simulink subsystem "PIDFeedFowardDigital_SubSystem"  (R2020b)
settings: Solver=VariableStepAuto  StartTime=0.0  StopTime=10.0  RelTol=1e-3
values from neighbouring files (symbols this model uses):
  Beq = BeqEst    [loadParNominal.m]
  Jeq = mot.J+(mld.J/gbox.N1^2)    [loadParNominal.m]
  Req = mot.R + sens.curr.Rs    [loadParNominal.m]
undefined symbols (not defined in the file or in its folder): drv, gbox, mld, mot
settings Model: Creator=umbe  LastModifiedBy=umbe

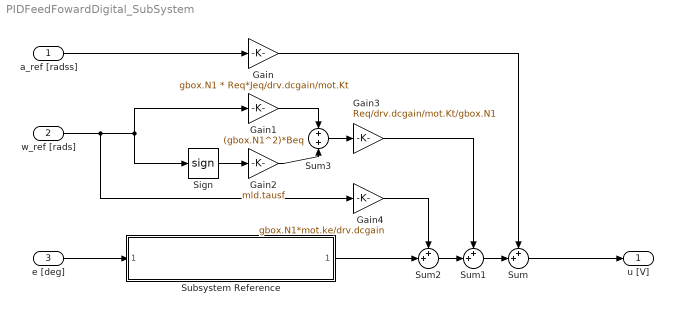
== system PIDFeedFowardDigital_SubSystem ==
  a_ref [radss] : Inport
  w_ref [rads] : Inport  Port=2
  e [deg] : Inport  Port=3
  Gain : Gain  Gain=gbox.N1 * Req*Jeq/drv.dcgain/mot.Kt
  Gain1 : Gain  Gain=(gbox.N1^2)*Beq
  Gain2 : Gain  Gain=mld.tausf
  Gain3 : Gain  Gain=Req/drv.dcgain/mot.Kt/gbox.N1
  Gain4 : Gain  Gain=gbox.N1*mot.ke/drv.dcgain
  Sign : Signum
  Subsystem Reference : Subsystem  ReferencedSubsystem=PIDAntiWindupDigital_SubSystem
  Sum : Sum  Inputs=++|
  Sum1 : Sum  Inputs=++|
  Sum2 : Sum  Inputs=++|
  Sum3 : Sum  Inputs=+|+
  u [V] : Outport
  wires:
  Sum2/1 -> Sum1/2
  Gain4/1 -> Sum2/1
  Sum1/1 -> Sum/2
  Gain3/1 -> Sum1/1
  Gain1/1 -> Sum3/1
  Gain2/1 -> Sum3/2
  Sum3/1 -> Gain3/1
  Subsystem Reference/1 -> Sum2/2
  Sign/1 -> Gain2/1
  w_ref [rads]/1 -> Gain1/1, Sign/1, Gain4/1
  Gain/1 -> Sum/1
  Sum/1 -> u [V]/1
  a_ref [radss]/1 -> Gain/1
  e [deg]/1 -> Subsystem Reference/1
